simulink model "plant_with_pi_to_pdf"  (R2015b)
settings: Solver=VariableStepAuto  StartTime=0.0  StopTime=10.0  RelTol=1e-3
undefined symbols (not defined in the file): Den, Iq, Ki, Kp, Num
settings Model: Creator=Morten  LastModifiedBy=Morten

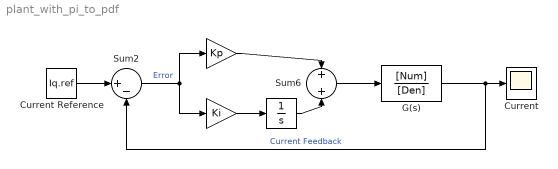
== system plant_with_pi_to_pdf ==
  " " : Integrator
  " " : Gain  Gain=Ki
  " " : Gain  Gain=Kp
  Current : Scope
  "Current Reference " : Constant  Value=Iq.ref
  G(s) : TransferFcn  Numerator=[Num]  Denominator=[Den]
  Sum2 : Sum  Inputs=|+-
  Sum6 : Sum
  wires:
  Sum2/1 -> " "/1, " "/1  "Error"
  "Current Reference "/1 -> Sum2/1
  G(s)/1 -> Sum2/2, Current/1  "Current Feedback"
  " "/1 -> Sum6/1
  " "/1 -> " "/1
  " "/1 -> Sum6/2
  Sum6/1 -> G(s)/1
